simulink model "mavsim_trim"  (Simulink 8.8)
settings: Solver=FixedStepAuto  StartTime=0.0  StopTime=inf  FixedStep=.005  RelTol=1e-3  EnableMultiTasking=on
InitFcn:
  | param_mavsim
undefined symbols (not defined in the file or in its folder): forces_moments, P
settings Model: SuppressorTable=22 serialization::archive 11 0 3 0 0 0 11 0  Creator=nmd89  LastModifiedBy=nmd89
settings DataIOCC: LimitDataPoints=off  SaveFormat=Dataset  SignalLoggingSaveFormat=Dataset
settings DebuggingCC: UnderspecifiedInitializationDetection=Simplified  MergeDetectMultiDrivingBlocksExec=error  FcnCallInpInsideContextMsg=error  StateNameClashWarn=none
settings HardwareCC: ProdBitPerPointer=64  ProdBitPerSizeT=64  ProdBitPerPtrDiffT=64  ProdLargestAtomicFloat=Float  ProdIntDivRoundTo=Zero  ProdEndianess=LittleEndian  ProdWordSize=64  ProdHWDeviceType=Intel->x86-64 (Windows64)
settings ModelReferenceCC: PropagateSignalLabelsOutOfModel=on
settings GRTTargetCC: CombineOutputUpdateFcns=on  GRTInterface=off

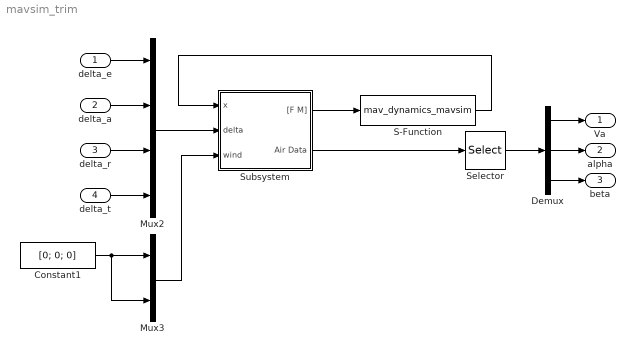
== system mavsim_trim ==
  delta_e : Inport
  delta_a : Inport  Port=2
  delta_r : Inport  Port=3
  delta_t : Inport  Port=4
  Constant1 : Constant  Value=[0; 0; 0]
  Demux : Demux  Outputs=3
  Mux2 : Mux
  Mux3 : Mux  Inputs=2
  S-Function : S-Function  FunctionName=mav_dynamics_mavsim  Parameters=P  SFunctionDeploymentMode=off  EnableBusSupport=off
  Selector : Selector  InputPortWidth=6  IndexOptions=Index vector (dialog)  Indices=[1 2 3]  OutputSizes=1
  Subsystem : Subsystem
  Va : Outport
  alpha : Outport  Port=2
  beta : Outport  Port=3
  wires:
  S-Function/1 -> Subsystem/1(x)
  Constant1/1 -> Mux3/2, Mux3/1
  Subsystem/1("[F M]") -> S-Function/1
  Mux2/1 -> Subsystem/2(delta)
  delta_e/1 -> Mux2/1
  delta_a/1 -> Mux2/2
  delta_r/1 -> Mux2/3
  delta_t/1 -> Mux2/4
  Mux3/1 -> Subsystem/3(wind)
  Subsystem/2(Air Data) -> Selector/1
  Selector/1 -> Demux/1
  Demux/1 -> Va/1
  Demux/2 -> alpha/1
  Demux/3 -> beta/1

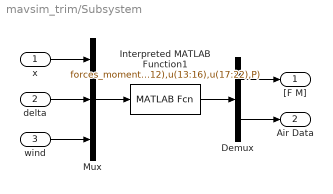
== system mavsim_trim/Subsystem ==
  x : Inport
  delta : Inport  Port=2
  wind : Inport  Port=3
  Demux : Demux  Outputs=[6;6]
  Interpreted MATLAB Function1 : MATLABFcn  MATLABFcn=forces_moments(u(1:12),u(13:16),u(17:22),P)
  Mux : Mux  Inputs=3
  "[F M]" : Outport
  Air Data : Outport  Port=2
  wires:
  Mux/1 -> Interpreted MATLAB Function1/1
  Interpreted MATLAB Function1/1 -> Demux/1
  Demux/1 -> "[F M]"/1
  Demux/2 -> Air Data/1
  x/1 -> Mux/1
  delta/1 -> Mux/2
  wind/1 -> Mux/3
